simulink model "Throttle_Position_Sensor_Model"  (R2023a)
settings: Solver=VariableStepAuto  StartTime=0.0  StopTime=10.0  RelTol=1e-3
libraries: simulink x1
settings Model: Creator=ItShop  LastModifiedBy=ItShop

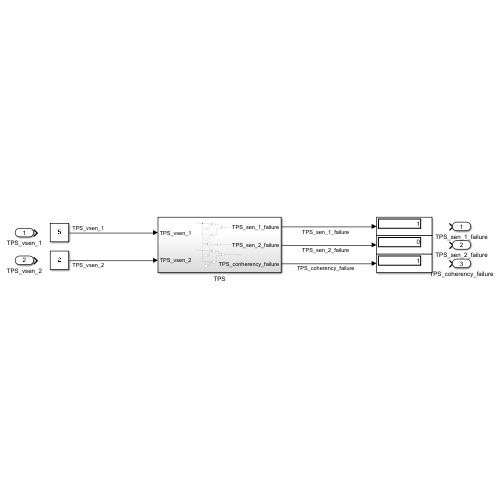
[thumbnail: Simulink's stored preview of the top-level diagram]
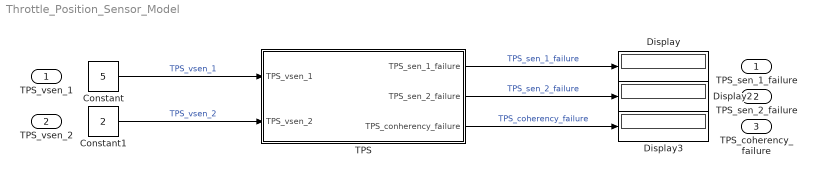
== system Throttle_Position_Sensor_Model ==
  TPS_vsen_1 : Inport  OutDataTypeStr=single
  TPS_vsen_2 : Inport  Port=2  OutDataTypeStr=single
  Constant : Constant  Value=5  OutDataTypeStr=single
  Constant1 : Constant  Value=2  OutDataTypeStr=single
  Display : Display
  Display2 : Display
  Display3 : Display
  TPS : Subsystem
  TPS_sen_1_failure : Outport  OutDataTypeStr=boolean
  TPS_sen_2_failure : Outport  Port=2  OutDataTypeStr=boolean
  TPS_coherency_failure : Outport  Port=3  OutDataTypeStr=boolean
  wires:
  Constant1/1 -> TPS/2(TPS_vsen_2)  "TPS_vsen_2"
  Constant/1 -> TPS/1(TPS_vsen_1)  "TPS_vsen_1"
  TPS/1(TPS_sen_1_failure) -> Display/1  "TPS_sen_1_failure"
  TPS/3(TPS_conherency_failure) -> Display3/1  "TPS_coherency_failure"
  TPS/2(TPS_sen_2_failure) -> Display2/1  "TPS_sen_2_failure"

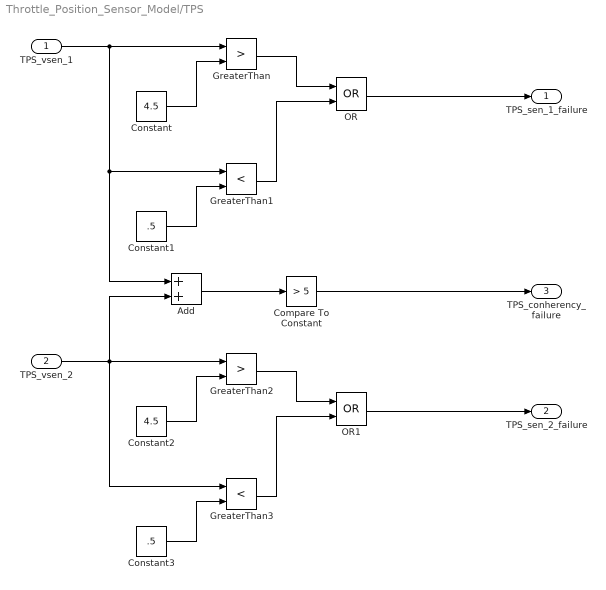
== system Throttle_Position_Sensor_Model/TPS ==
  TPS_vsen_1 : Inport  OutDataTypeStr=single
  TPS_vsen_2 : Inport  Port=2  OutDataTypeStr=single
  Add : Sum
  Compare To Constant : simulink/Logic and Bit Operations/Compare To Constant  relop=>  const=5  OutDataTypeStr=boolean
  Constant : Constant  Value=4.5
  Constant1 : Constant  Value=.5
  Constant2 : Constant  Value=4.5
  Constant3 : Constant  Value=.5
  GreaterThan : RelationalOperator  Operator=>  OutDataTypeStr=boolean  RndMeth=Simplest  InputSameDT=off
  GreaterThan1 : RelationalOperator  Operator=<  OutDataTypeStr=boolean  RndMeth=Simplest  InputSameDT=off
  GreaterThan2 : RelationalOperator  Operator=>  OutDataTypeStr=boolean  RndMeth=Simplest  InputSameDT=off
  GreaterThan3 : RelationalOperator  Operator=<  OutDataTypeStr=boolean  RndMeth=Simplest  InputSameDT=off
  OR : Logic  Operator=OR  AllPortsSameDT=off  OutDataTypeStr=boolean
  OR1 : Logic  Operator=OR  AllPortsSameDT=off  OutDataTypeStr=boolean
  TPS_sen_1_failure : Outport  OutDataTypeStr=boolean
  TPS_sen_2_failure : Outport  Port=2  OutDataTypeStr=boolean
  TPS_conherency_failure : Outport  Port=3  OutDataTypeStr=boolean
  wires:
  TPS_vsen_1/1 -> Add/1, GreaterThan1/1, GreaterThan/1
  Constant/1 -> GreaterThan/2
  Constant1/1 -> GreaterThan1/2
  GreaterThan/1 -> OR/1
  GreaterThan1/1 -> OR/2
  OR/1 -> TPS_sen_1_failure/1
  OR1/1 -> TPS_sen_2_failure/1
  GreaterThan3/1 -> OR1/2
  GreaterThan2/1 -> OR1/1
  Constant3/1 -> GreaterThan3/2
  Constant2/1 -> GreaterThan2/2
  TPS_vsen_2/1 -> Add/2, GreaterThan2/1, GreaterThan3/1
  Add/1 -> Compare To Constant/1
  Compare To Constant/1 -> TPS_conherency_failure/1
